simulink model "SSRFFT_basic_test"  (R2019b)
settings: Solver=VariableStepAuto  StartTime=0.0  StopTime=1024*2  RelTol=1e-3
libraries: xbsIndex_r4 x6, xrbsSSR_Library x5
settings Model: Creator=jpsmith  LastModifiedBy=jpsmith
settings DataIOCC: ReturnWorkspaceOutputs=off
settings DebuggingCC: ArithmeticOperatorsInVariantConditions=warning
settings SFSimCC: CustomCodeUndefinedFunction=UseInterfaceOnly

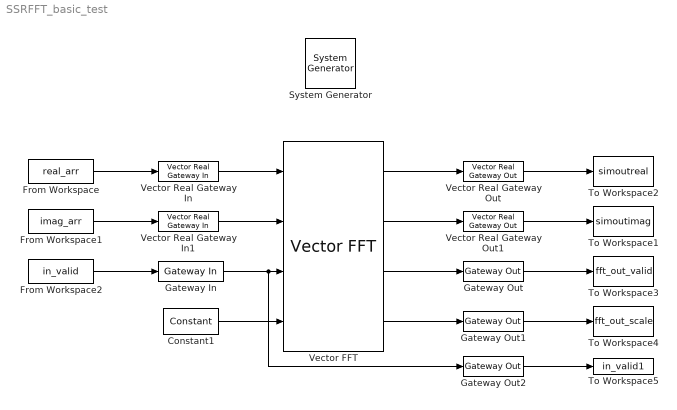
== system SSRFFT_basic_test ==
  " System Generator" : xbsIndex_r4/ System Generator  Tag=genX  xilinxfamily=zynquplusRFSOC  part=xczu28dr  speed=-2-e  package=ffvg1517  synthesis_tool=Vivado  clock_wrapper=Clock Enables  directory=./netlist  proj_type=Vivado  Synth_file=Vivado Synthesis Defaults  Impl_file=Vivado Implementation Defaults  testbench=off  simulink_period=1  sysclk_period=10  dcm_input_clock_period=10  incr_netlist=off  trim_vbits=Everywhere in SubSystem  dbl_ovrd=According to Block Masks  core_generation=According to Block Masks  run_coregen=off  deprecated_control=off  eval_field=0  block_type=sysgen
  Constant1 : xbsIndex_r4/Constant  const=0  gui_display_data_type=Fixed-point  arith_type=Signed (2's comp)  n_bits=10  bin_pt=0  preci_type=Single  exp_width=8  frac_width=24  explicit_period=on  period=1  equ=P=C  opselect=C  inp2=PCIN>>17  opr=+  inp1=P  carry=CIN  dbl_ovrd=off  block_type=constant
  From Workspace : FromWorkspace  VariableName=real_arr  OutDataTypeStr=double  SampleTime=1  Interpolate=off  OutputAfterFinalValue=Setting to zero
  From Workspace1 : FromWorkspace  VariableName=imag_arr  OutDataTypeStr=double  SampleTime=1  Interpolate=off  OutputAfterFinalValue=Setting to zero
  From Workspace2 : FromWorkspace  VariableName=in_valid  SampleTime=1  OutputAfterFinalValue=Setting to zero
  Gateway In : xbsIndex_r4/Gateway In  gui_display_data_type=Boolean  arith_type=Boolean  n_bits=16  bin_pt=14  preci_type=Single  exp_width=8  frac_width=24  rows=1  columns=1  quantization="Round  (unbiased: +/- Inf)"  overflow=Saturate  period=1  UseAsADC=off  ADCChannel='1'  interface=None  automatic_assignment=on  address_offset=hex2dec('00')  intf_name=''  intf_description=''  default_value=0  timing_constraint=None  locs_specified=off  LOCs={}  io_standard={}  inherit_from_input=off  hdl_port=on  dbl_ovrd=off  block_type=gatewayin
  Gateway Out : xbsIndex_r4/Gateway Out  inherit_from_input=on  hdl_port=on  rows=1  columns=1  UseAsDAC=off  DACChannel='1'  interface=None  automatic_assignment=on  address_offset=hex2dec('00')  intf_name=''  intf_description=''  timing_constraint=None  locs_specified=off  LOCs={}  io_standard={}  block_type=gatewayout
  Gateway Out1 : xbsIndex_r4/Gateway Out  inherit_from_input=on  hdl_port=on  rows=1  columns=1  UseAsDAC=off  DACChannel='1'  interface=None  automatic_assignment=on  address_offset=hex2dec('00')  intf_name=''  intf_description=''  timing_constraint=None  locs_specified=off  LOCs={}  io_standard={}  block_type=gatewayout
  Gateway Out2 : xbsIndex_r4/Gateway Out  inherit_from_input=on  hdl_port=on  rows=1  columns=1  UseAsDAC=off  DACChannel='1'  interface=None  automatic_assignment=on  address_offset=hex2dec('00')  intf_name=''  intf_description=''  timing_constraint=None  locs_specified=off  LOCs={}  io_standard={}  block_type=gatewayout
  To Workspace1 : ToWorkspace  VariableName=simoutimag  SampleTime=-1
      settings: Save2DSignal=2-D array (concatenate along first dimension)
  To Workspace2 : ToWorkspace  VariableName=simoutreal  SampleTime=-1
      settings: Save2DSignal=2-D array (concatenate along first dimension)
  To Workspace3 : ToWorkspace  VariableName=fft_out_valid  SaveFormat=Timeseries  SampleTime=-1
      settings: Save2DSignal=2-D array (concatenate along first dimension)
  To Workspace4 : ToWorkspace  VariableName=fft_out_scale  SaveFormat=Timeseries  SampleTime=-1
      settings: Save2DSignal=2-D array (concatenate along first dimension)
  To Workspace5 : ToWorkspace  VariableName=in_valid1  SaveFormat=Timeseries  SampleTime=-1
      settings: Save2DSignal=2-D array (concatenate along first dimension)
  Vector FFT : xrbsSSR_Library/Vector FFT  sg_ssr=4  N=1024  W_high=1  W_low=-17  n_bits=18  bin_pt=17  bram_threshold=258  block_type=fft_ssr
      settings: SourceProductName=Xilinx SSR Blockset
  Vector Real Gateway In : xrbsSSR_Library/Vector Real Gateway In  gui_display_data_type=Fixed-point  arith_type="Signed  (2's comp)"  n_bits=16  bin_pt=15  preci_type=Single  exp_width=8  frac_width=24  quantization="Round  (unbiased: +/- Inf)"  overflow=Saturate  period=1  sg_ssr=4  sg_ssr_prev=4  UseAsADC=off  ADCChannel='1'  interface=None  interface_prev=1  automatic_assignment=off  address_offset=hex2dec('00')  intf_name=''  intf_description=''  default_value=0  timing_constraint=None  locs_specified=off  LOCs={}  io_standard={}  hdl_port=on  dbl_ovrd=off  block_type=realgatewayin_ssr  name_prev=Vector Real Gateway In
      settings: SourceProductName=Xilinx SSR Blockset  infoedit=The Vector Real Gateway in block converts Vector inputs of type Simulink integer, single, double and fixed-point to Xilinx fixed-point or floating-point data type.<br><br>Hardware notes: In hardware these blocks become top level input ports.
  Vector Real Gateway In1 : xrbsSSR_Library/Vector Real Gateway In  gui_display_data_type=Fixed-point  arith_type="Signed  (2's comp)"  n_bits=16  bin_pt=15  preci_type=Single  exp_width=8  frac_width=24  quantization="Round  (unbiased: +/- Inf)"  overflow=Saturate  period=1  sg_ssr=4  sg_ssr_prev=4  UseAsADC=off  ADCChannel='1'  interface=None  interface_prev=1  automatic_assignment=off  address_offset=hex2dec('00')  intf_name=''  intf_description=''  default_value=0  timing_constraint=None  locs_specified=off  LOCs={}  io_standard={}  hdl_port=on  dbl_ovrd=off  block_type=realgatewayin_ssr  name_prev=Vector Real Gateway In1
      settings: SourceProductName=Xilinx SSR Blockset  infoedit=The Vector Real Gateway in block converts Vector inputs of type Simulink integer, single, double and fixed-point to Xilinx fixed-point or floating-point data type.<br><br>Hardware notes: In hardware these blocks become top level input ports.
  Vector Real Gateway Out : xrbsSSR_Library/Vector Real Gateway Out  inherit_from_input=off  hdl_port=on  rows=1  columns=1  UseAsDAC=off  DACChannel='1'  interface=None  automatic_assignment=on  address_offset=hex2dec('00')  intf_name=''  intf_description=''  timing_constraint=None  locs_specified=off  LOCs={}  io_standard={}  block_type=realgatewayout_ssr  sg_ssr=4  sg_ssr_prev=4  sg_ssr_name=vect_real_gwayout  name_prev=Vector Real Gateway Out
      settings: SourceProductName=Xilinx SSR Blockset  infoedit=The Vector Real Gateway out block converts Xilinx fixed-point or floating-point type vector inputs into vector ouputs of type Simulink integer, single, double, or fixed-point.<br><br>Hardware notes: In hardware these blocks become top level output ports or are discarded, depending on how they are configured.
  Vector Real Gateway Out1 : xrbsSSR_Library/Vector Real Gateway Out  inherit_from_input=off  hdl_port=on  rows=1  columns=1  UseAsDAC=off  DACChannel='1'  interface=None  automatic_assignment=on  address_offset=hex2dec('00')  intf_name=''  intf_description=''  timing_constraint=None  locs_specified=off  LOCs={}  io_standard={}  block_type=realgatewayout_ssr  sg_ssr=4  sg_ssr_prev=4  sg_ssr_name=vect_real_gwayout  name_prev=Vector Real Gateway Out1
      settings: SourceProductName=Xilinx SSR Blockset  infoedit=The Vector Real Gateway out block converts Xilinx fixed-point or floating-point type vector inputs into vector ouputs of type Simulink integer, single, double, or fixed-point.<br><br>Hardware notes: In hardware these blocks become top level output ports or are discarded, depending on how they are configured.
  wires:
  Vector Real Gateway Out/1 -> To Workspace2/1
  From Workspace/1 -> Vector Real Gateway In/1
  From Workspace1/1 -> Vector Real Gateway In1/1
  Vector Real Gateway Out1/1 -> To Workspace1/1
  Vector Real Gateway In/1 -> Vector FFT/1
  Vector Real Gateway In1/1 -> Vector FFT/2
  Vector FFT/1 -> Vector Real Gateway Out/1
  Vector FFT/2 -> Vector Real Gateway Out1/1
  Gateway Out1/1 -> To Workspace4/1
  Gateway Out/1 -> To Workspace3/1
  Vector FFT/3 -> Gateway Out/1
  Vector FFT/4 -> Gateway Out1/1
  Constant1/1 -> Vector FFT/4
  From Workspace2/1 -> Gateway In/1
  Gateway In/1 -> Gateway Out2/1, Vector FFT/3
  Gateway Out2/1 -> To Workspace5/1
